simulink model "Train_Model"  (R2023b)
settings: Solver=VariableStepAuto  StartTime=0.0  StopTime=10.0  RelTol=1e-3
undefined symbols (not defined in the file or in its folder): g, k, M1, M2, mu
settings Model: Creator=sayeholoumi  LastModifiedBy=sayeholoumi

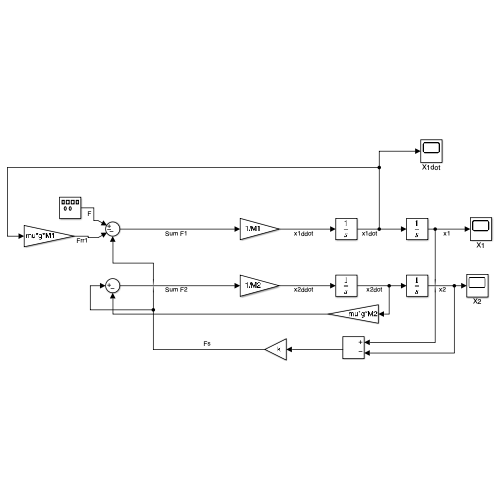
[thumbnail: Simulink's stored preview of the top-level diagram]
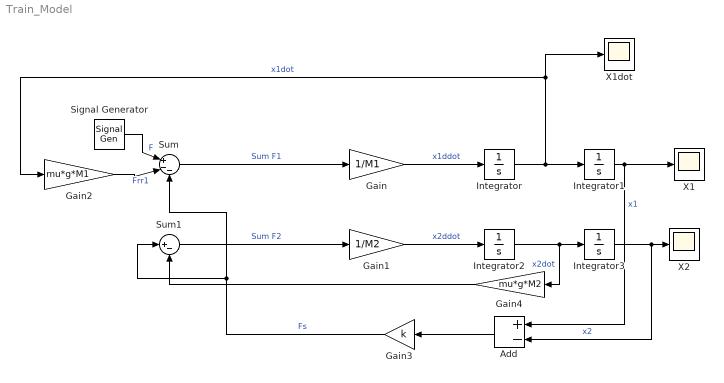
== system Train_Model ==
  Add : Sum  Inputs=+-
  Gain : Gain  Gain=1/M1
  Gain1 : Gain  Gain=1/M2
  Gain2 : Gain  Gain=mu*g*M1
  Gain3 : Gain  Gain=k
  Gain4 : Gain  Gain=mu*g*M2
  Integrator{,1..3} (4 alike) : Integrator
  Signal Generator : SignalGenerator  Units=rad/sec
  Sum : Sum  Inputs=|+--
  Sum1 : Sum  Inputs=|+-
  X1 : Scope
  X1dot : Scope
  X2 : Scope
  wires:
  Sum/1 -> Gain/1  "Sum F1"
  Sum1/1 -> Gain1/1  "Sum F2"
  Gain/1 -> Integrator/1  "x1ddot"
  Integrator/1 -> X1dot/1, Gain2/1, Integrator1/1  "x1dot"
  Gain1/1 -> Integrator2/1  "x2ddot"
  Integrator2/1 -> Gain4/1, Integrator3/1  "x2dot"
  Integrator1/1 -> Add/1, X1/1  "x1"
  Integrator3/1 -> Add/2, X2/1  "x2"
  Signal Generator/1 -> Sum/1  "F"
  Gain2/1 -> Sum/2  "Frr1"
  Add/1 -> Gain3/1
  Gain3/1 -> Sum1/1, Sum/3  "Fs"
  Gain4/1 -> Sum1/2
